simulink subsystem "PROGRAM_COUNTER_06_SS"  (R2022a)
settings: Solver=VariableStepAuto  StartTime=0.0  StopTime=10.0  RelTol=1e-3
libraries: hdlBasic x1928, hlsBasic x1
(part 8 of 12)

== system PROGRAM_COUNTER_06_SS/SUMADOR_64_BITS_00/ALU_SUM_7 ==
  CARRY_IN (1 BIT) : Inport
  A_INPUT (1 BIT) : Inport  Port=2
  B_INPUT (1 BIT) : Inport  Port=3
  Inverter1 : hdlBasic/Inverter  en=off  latency=0  XmcBlockStatus=1  maskContainerNames=group2  block_type=inv  block_config=sysgen:Inverter_config
  Inverter8 : hdlBasic/Inverter  en=off  latency=0  XmcBlockStatus=1  maskContainerNames=group2  block_type=inv  block_config=sysgen:Inverter_config
  Inverter9 : hdlBasic/Inverter  en=off  latency=0  XmcBlockStatus=1  maskContainerNames=group2  block_type=inv  block_config=sysgen:Inverter_config
  Logical : hdlBasic/Logical  logical_function=AND  inputs=2  en=off  latency=0  precision=Full  arith_type=Unsigned  n_bits=16  bin_pt=0  align_bp=on  overflow=[]  quantization=[]  XmcBlockStatus=1  maskContainerNames=tabcontainer1  block_type=logical  block_config=sysgen:Logical_config
  Logical1 : hdlBasic/Logical  logical_function=AND  inputs=2  en=off  latency=0  precision=Full  arith_type=Unsigned  n_bits=16  bin_pt=0  align_bp=on  overflow=[]  quantization=[]  XmcBlockStatus=1  maskContainerNames=tabcontainer1  block_type=logical  block_config=sysgen:Logical_config
  Logical2 : hdlBasic/Logical  logical_function=AND  inputs=2  en=off  latency=0  precision=Full  arith_type=Unsigned  n_bits=16  bin_pt=0  align_bp=on  overflow=[]  quantization=[]  XmcBlockStatus=1  maskContainerNames=tabcontainer1  block_type=logical  block_config=sysgen:Logical_config
  Logical{4..6,9} (4 alike) : hdlBasic/Logical  logical_function=AND  inputs=3  en=off  latency=0  precision=Full  arith_type=Unsigned  n_bits=16  bin_pt=0  align_bp=on  overflow=[]  quantization=[]  XmcBlockStatus=1  maskContainerNames=tabcontainer1  block_type=logical  block_config=sysgen:Logical_config
  Sum : hdlBasic/Logical  logical_function=OR  inputs=4  en=off  latency=0  precision=Full  arith_type=Unsigned  n_bits=16  bin_pt=0  align_bp=on  overflow=[]  quantization=[]  XmcBlockStatus=1  maskContainerNames=tabcontainer1  block_type=logical  block_config=sysgen:Logical_config
  c_out : hdlBasic/Logical  logical_function=OR  inputs=3  en=off  latency=0  precision=Full  arith_type=Unsigned  n_bits=16  bin_pt=0  align_bp=on  overflow=[]  quantization=[]  XmcBlockStatus=1  maskContainerNames=tabcontainer1  block_type=logical  block_config=sysgen:Logical_config
  ALU_OUT (1 BIT) : Outport
  CARRY_OUT (1 BIT) : Outport  Port=2
  wires:
  c_out/1 -> CARRY_OUT (1 BIT)/1
  Logical2/1 -> c_out/3
  Sum/1 -> ALU_OUT (1 BIT)/1
  Inverter9/1 -> Logical4/3, Logical9/3
  Logical5/1 -> Sum/4
  Logical/1 -> c_out/1
  Logical4/1 -> Sum/1
  Logical9/1 -> Sum/2
  Logical6/1 -> Sum/3
  Inverter1/1 -> Logical9/1, Logical6/1
  B_INPUT (1 BIT)/1 -> Inverter9/1, Logical2/2, Logical1/2, Logical6/3, Logical5/3
  CARRY_IN (1 BIT)/1 -> Logical/1, Logical1/1, Logical4/1, Logical5/1, Inverter1/1
  Inverter8/1 -> Logical4/2, Logical6/2
  Logical1/1 -> c_out/2
  A_INPUT (1 BIT)/1 -> Logical9/2, Logical2/1, Logical/2, Logical5/2, Inverter8/1

== system PROGRAM_COUNTER_06_SS/SUMADOR_64_BITS_00/ALU_SUM_8 ==
  CARRY_IN (1 BIT) : Inport
  A_INPUT (1 BIT) : Inport  Port=2
  B_INPUT (1 BIT) : Inport  Port=3
  Inverter1 : hdlBasic/Inverter  en=off  latency=0  XmcBlockStatus=1  maskContainerNames=group2  block_type=inv  block_config=sysgen:Inverter_config
  Inverter8 : hdlBasic/Inverter  en=off  latency=0  XmcBlockStatus=1  maskContainerNames=group2  block_type=inv  block_config=sysgen:Inverter_config
  Inverter9 : hdlBasic/Inverter  en=off  latency=0  XmcBlockStatus=1  maskContainerNames=group2  block_type=inv  block_config=sysgen:Inverter_config
  Logical : hdlBasic/Logical  logical_function=AND  inputs=2  en=off  latency=0  precision=Full  arith_type=Unsigned  n_bits=16  bin_pt=0  align_bp=on  overflow=[]  quantization=[]  XmcBlockStatus=1  maskContainerNames=tabcontainer1  block_type=logical  block_config=sysgen:Logical_config
  Logical1 : hdlBasic/Logical  logical_function=AND  inputs=2  en=off  latency=0  precision=Full  arith_type=Unsigned  n_bits=16  bin_pt=0  align_bp=on  overflow=[]  quantization=[]  XmcBlockStatus=1  maskContainerNames=tabcontainer1  block_type=logical  block_config=sysgen:Logical_config
  Logical2 : hdlBasic/Logical  logical_function=AND  inputs=2  en=off  latency=0  precision=Full  arith_type=Unsigned  n_bits=16  bin_pt=0  align_bp=on  overflow=[]  quantization=[]  XmcBlockStatus=1  maskContainerNames=tabcontainer1  block_type=logical  block_config=sysgen:Logical_config
  Logical{4..6,9} (4 alike) : hdlBasic/Logical  logical_function=AND  inputs=3  en=off  latency=0  precision=Full  arith_type=Unsigned  n_bits=16  bin_pt=0  align_bp=on  overflow=[]  quantization=[]  XmcBlockStatus=1  maskContainerNames=tabcontainer1  block_type=logical  block_config=sysgen:Logical_config
  Sum : hdlBasic/Logical  logical_function=OR  inputs=4  en=off  latency=0  precision=Full  arith_type=Unsigned  n_bits=16  bin_pt=0  align_bp=on  overflow=[]  quantization=[]  XmcBlockStatus=1  maskContainerNames=tabcontainer1  block_type=logical  block_config=sysgen:Logical_config
  c_out : hdlBasic/Logical  logical_function=OR  inputs=3  en=off  latency=0  precision=Full  arith_type=Unsigned  n_bits=16  bin_pt=0  align_bp=on  overflow=[]  quantization=[]  XmcBlockStatus=1  maskContainerNames=tabcontainer1  block_type=logical  block_config=sysgen:Logical_config
  ALU_OUT (1 BIT) : Outport
  CARRY_OUT (1 BIT) : Outport  Port=2
  wires:
  c_out/1 -> CARRY_OUT (1 BIT)/1
  Logical2/1 -> c_out/3
  Sum/1 -> ALU_OUT (1 BIT)/1
  Inverter9/1 -> Logical4/3, Logical9/3
  Logical5/1 -> Sum/4
  Logical/1 -> c_out/1
  Logical4/1 -> Sum/1
  Logical9/1 -> Sum/2
  Logical6/1 -> Sum/3
  Inverter1/1 -> Logical9/1, Logical6/1
  B_INPUT (1 BIT)/1 -> Inverter9/1, Logical2/2, Logical1/2, Logical6/3, Logical5/3
  CARRY_IN (1 BIT)/1 -> Logical/1, Logical1/1, Logical4/1, Logical5/1, Inverter1/1
  Inverter8/1 -> Logical4/2, Logical6/2
  Logical1/1 -> c_out/2
  A_INPUT (1 BIT)/1 -> Logical9/2, Logical2/1, Logical/2, Logical5/2, Inverter8/1

== system PROGRAM_COUNTER_06_SS/SUMADOR_64_BITS_00/ALU_SUM_9 ==
  CARRY_IN (1 BIT) : Inport
  A_INPUT (1 BIT) : Inport  Port=2
  B_INPUT (1 BIT) : Inport  Port=3
  Inverter1 : hdlBasic/Inverter  en=off  latency=0  XmcBlockStatus=1  maskContainerNames=group2  block_type=inv  block_config=sysgen:Inverter_config
  Inverter8 : hdlBasic/Inverter  en=off  latency=0  XmcBlockStatus=1  maskContainerNames=group2  block_type=inv  block_config=sysgen:Inverter_config
  Inverter9 : hdlBasic/Inverter  en=off  latency=0  XmcBlockStatus=1  maskContainerNames=group2  block_type=inv  block_config=sysgen:Inverter_config
  Logical : hdlBasic/Logical  logical_function=AND  inputs=2  en=off  latency=0  precision=Full  arith_type=Unsigned  n_bits=16  bin_pt=0  align_bp=on  overflow=[]  quantization=[]  XmcBlockStatus=1  maskContainerNames=tabcontainer1  block_type=logical  block_config=sysgen:Logical_config
  Logical1 : hdlBasic/Logical  logical_function=AND  inputs=2  en=off  latency=0  precision=Full  arith_type=Unsigned  n_bits=16  bin_pt=0  align_bp=on  overflow=[]  quantization=[]  XmcBlockStatus=1  maskContainerNames=tabcontainer1  block_type=logical  block_config=sysgen:Logical_config
  Logical2 : hdlBasic/Logical  logical_function=AND  inputs=2  en=off  latency=0  precision=Full  arith_type=Unsigned  n_bits=16  bin_pt=0  align_bp=on  overflow=[]  quantization=[]  XmcBlockStatus=1  maskContainerNames=tabcontainer1  block_type=logical  block_config=sysgen:Logical_config
  Logical{4..6,9} (4 alike) : hdlBasic/Logical  logical_function=AND  inputs=3  en=off  latency=0  precision=Full  arith_type=Unsigned  n_bits=16  bin_pt=0  align_bp=on  overflow=[]  quantization=[]  XmcBlockStatus=1  maskContainerNames=tabcontainer1  block_type=logical  block_config=sysgen:Logical_config
  Sum : hdlBasic/Logical  logical_function=OR  inputs=4  en=off  latency=0  precision=Full  arith_type=Unsigned  n_bits=16  bin_pt=0  align_bp=on  overflow=[]  quantization=[]  XmcBlockStatus=1  maskContainerNames=tabcontainer1  block_type=logical  block_config=sysgen:Logical_config
  c_out : hdlBasic/Logical  logical_function=OR  inputs=3  en=off  latency=0  precision=Full  arith_type=Unsigned  n_bits=16  bin_pt=0  align_bp=on  overflow=[]  quantization=[]  XmcBlockStatus=1  maskContainerNames=tabcontainer1  block_type=logical  block_config=sysgen:Logical_config
  ALU_OUT (1 BIT) : Outport
  CARRY_OUT (1 BIT) : Outport  Port=2
  wires:
  c_out/1 -> CARRY_OUT (1 BIT)/1
  Logical2/1 -> c_out/3
  Sum/1 -> ALU_OUT (1 BIT)/1
  Inverter9/1 -> Logical4/3, Logical9/3
  Logical5/1 -> Sum/4
  Logical/1 -> c_out/1
  Logical4/1 -> Sum/1
  Logical9/1 -> Sum/2
  Logical6/1 -> Sum/3
  Inverter1/1 -> Logical9/1, Logical6/1
  B_INPUT (1 BIT)/1 -> Inverter9/1, Logical2/2, Logical1/2, Logical6/3, Logical5/3
  CARRY_IN (1 BIT)/1 -> Logical/1, Logical1/1, Logical4/1, Logical5/1, Inverter1/1
  Inverter8/1 -> Logical4/2, Logical6/2
  Logical1/1 -> c_out/2
  A_INPUT (1 BIT)/1 -> Logical9/2, Logical2/1, Logical/2, Logical5/2, Inverter8/1

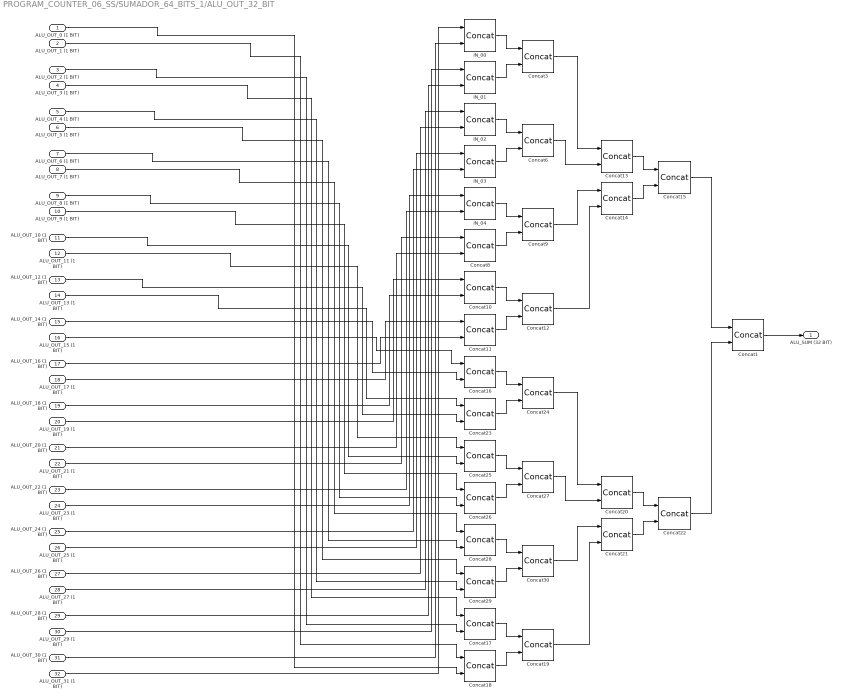
== system PROGRAM_COUNTER_06_SS/SUMADOR_64_BITS_1/ALU_OUT_32_BIT ==
  ALU_OUT_0 (1 BIT) : Inport
  ALU_OUT_1 (1 BIT) : Inport  Port=2
  ALU_OUT_2 (1 BIT) : Inport  Port=3
  ALU_OUT_3 (1 BIT) : Inport  Port=4
  ALU_OUT_4 (1 BIT) : Inport  Port=5
  ALU_OUT_5 (1 BIT) : Inport  Port=6
  ALU_OUT_6 (1 BIT) : Inport  Port=7
  ALU_OUT_7 (1 BIT) : Inport  Port=8
  ALU_OUT_8 (1 BIT) : Inport  Port=9
  ALU_OUT_9 (1 BIT) : Inport  Port=10
  ALU_OUT_10 (1 BIT) : Inport  Port=11
  ALU_OUT_11 (1 BIT) : Inport  Port=12
  ALU_OUT_12 (1 BIT) : Inport  Port=13
  ALU_OUT_13 (1 BIT) : Inport  Port=14
  ALU_OUT_14 (1 BIT) : Inport  Port=15
  ALU_OUT_15 (1 BIT) : Inport  Port=16
  ALU_OUT_16 (1 BIT) : Inport  Port=17
  ALU_OUT_17 (1 BIT) : Inport  Port=18
  ALU_OUT_18 (1 BIT) : Inport  Port=19
  ALU_OUT_19 (1 BIT) : Inport  Port=20
  ALU_OUT_20 (1 BIT) : Inport  Port=21
  ALU_OUT_21 (1 BIT) : Inport  Port=22
  ALU_OUT_22 (1 BIT) : Inport  Port=23
  ALU_OUT_23 (1 BIT) : Inport  Port=24
  ALU_OUT_24 (1 BIT) : Inport  Port=25
  ALU_OUT_25 (1 BIT) : Inport  Port=26
  ALU_OUT_26 (1 BIT) : Inport  Port=27
  ALU_OUT_27 (1 BIT) : Inport  Port=28
  ALU_OUT_28 (1 BIT) : Inport  Port=29
  ALU_OUT_29 (1 BIT) : Inport  Port=30
  ALU_OUT_30 (1 BIT) : Inport  Port=31
  ALU_OUT_31 (1 BIT) : Inport  Port=32
  Concat{1,3,6,8..30} (26 alike) : hdlBasic/Concat  num_inputs=2  XmcBlockStatus=1  maskContainerNames=group1  block_type=concat  block_config=sysgen:Concat_config
  IN_00 : hdlBasic/Concat  num_inputs=2  XmcBlockStatus=1  maskContainerNames=group1  block_type=concat  block_config=sysgen:Concat_config
  IN_01 : hdlBasic/Concat  num_inputs=2  XmcBlockStatus=1  maskContainerNames=group1  block_type=concat  block_config=sysgen:Concat_config
  IN_02 : hdlBasic/Concat  num_inputs=2  XmcBlockStatus=1  maskContainerNames=group1  block_type=concat  block_config=sysgen:Concat_config
  IN_03 : hdlBasic/Concat  num_inputs=2  XmcBlockStatus=1  maskContainerNames=group1  block_type=concat  block_config=sysgen:Concat_config
  IN_04 : hdlBasic/Concat  num_inputs=2  XmcBlockStatus=1  maskContainerNames=group1  block_type=concat  block_config=sysgen:Concat_config
  ALU_SUM (32 BIT) : Outport
  wires:
  ALU_OUT_0 (1 BIT)/1 -> Concat18/2
  ALU_OUT_1 (1 BIT)/1 -> Concat18/1
  ALU_OUT_2 (1 BIT)/1 -> Concat17/2
  ALU_OUT_3 (1 BIT)/1 -> Concat17/1
  ALU_OUT_4 (1 BIT)/1 -> Concat29/2
  ALU_OUT_5 (1 BIT)/1 -> Concat29/1
  ALU_OUT_6 (1 BIT)/1 -> Concat28/2
  ALU_OUT_7 (1 BIT)/1 -> Concat28/1
  ALU_OUT_8 (1 BIT)/1 -> Concat26/2
  ALU_OUT_9 (1 BIT)/1 -> Concat26/1
  ALU_OUT_10 (1 BIT)/1 -> Concat25/2
  ALU_OUT_11 (1 BIT)/1 -> Concat25/1
  ALU_OUT_12 (1 BIT)/1 -> Concat23/2
  ALU_OUT_13 (1 BIT)/1 -> Concat23/1
  ALU_OUT_14 (1 BIT)/1 -> Concat16/2
  ALU_OUT_15 (1 BIT)/1 -> Concat16/1
  ALU_OUT_16 (1 BIT)/1 -> Concat11/2
  ALU_OUT_17 (1 BIT)/1 -> Concat11/1
  ALU_OUT_18 (1 BIT)/1 -> Concat10/2
  ALU_OUT_19 (1 BIT)/1 -> Concat10/1
  ALU_OUT_20 (1 BIT)/1 -> Concat8/2
  ALU_OUT_21 (1 BIT)/1 -> Concat8/1
  ALU_OUT_22 (1 BIT)/1 -> IN_04/2
  ALU_OUT_23 (1 BIT)/1 -> IN_04/1
  ALU_OUT_24 (1 BIT)/1 -> IN_03/2
  ALU_OUT_25 (1 BIT)/1 -> IN_03/1
  ALU_OUT_26 (1 BIT)/1 -> IN_02/2
  ALU_OUT_27 (1 BIT)/1 -> IN_02/1
  ALU_OUT_28 (1 BIT)/1 -> IN_01/2
  ALU_OUT_29 (1 BIT)/1 -> IN_01/1
  ALU_OUT_30 (1 BIT)/1 -> IN_00/2
  ALU_OUT_31 (1 BIT)/1 -> IN_00/1
  Concat1/1 -> ALU_SUM (32 BIT)/1
  Concat12/1 -> Concat14/2
  Concat14/1 -> Concat15/2
  IN_04/1 -> Concat9/1
  Concat8/1 -> Concat9/2
  Concat15/1 -> Concat1/1
  Concat9/1 -> Concat14/1
  IN_03/1 -> Concat6/2
  IN_02/1 -> Concat6/1
  Concat25/1 -> Concat27/1
  Concat18/1 -> Concat19/2
  Concat23/1 -> Concat24/2
  Concat16/1 -> Concat24/1
  Concat24/1 -> Concat20/1
  Concat30/1 -> Concat21/1
  Concat13/1 -> Concat15/1
  Concat6/1 -> Concat13/2
  Concat26/1 -> Concat27/2
  Concat17/1 -> Concat19/1
  Concat20/1 -> Concat22/1
  Concat3/1 -> Concat13/1
  IN_00/1 -> Concat3/1
  Concat21/1 -> Concat22/2
  Concat29/1 -> Concat30/2
  Concat11/1 -> Concat12/2
  Concat28/1 -> Concat30/1
  Concat22/1 -> Concat1/2
  Concat19/1 -> Concat21/2
  Concat27/1 -> Concat20/2
  Concat10/1 -> Concat12/1
  IN_01/1 -> Concat3/2

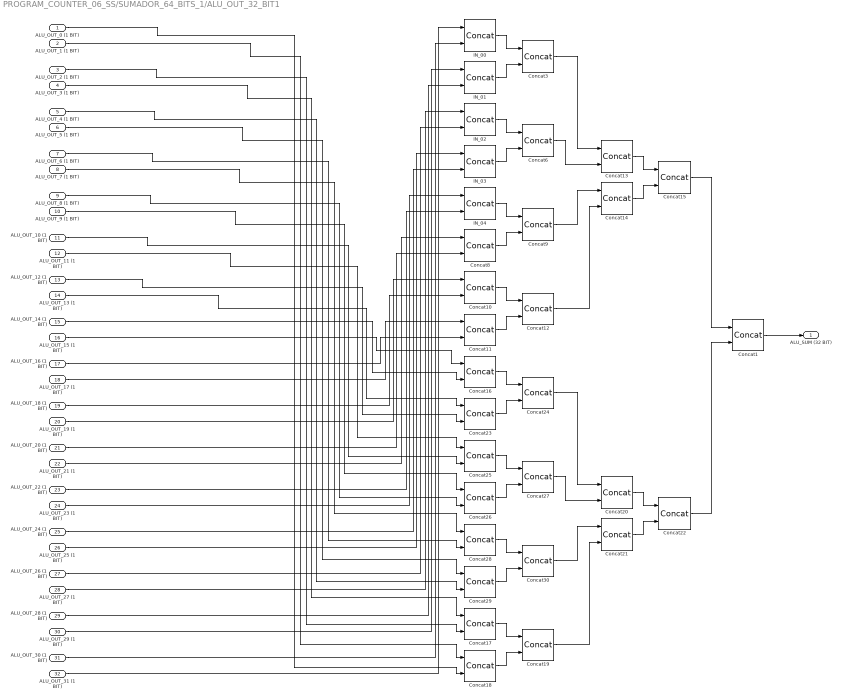
== system PROGRAM_COUNTER_06_SS/SUMADOR_64_BITS_1/ALU_OUT_32_BIT1 ==
  ALU_OUT_0 (1 BIT) : Inport
  ALU_OUT_1 (1 BIT) : Inport  Port=2
  ALU_OUT_2 (1 BIT) : Inport  Port=3
  ALU_OUT_3 (1 BIT) : Inport  Port=4
  ALU_OUT_4 (1 BIT) : Inport  Port=5
  ALU_OUT_5 (1 BIT) : Inport  Port=6
  ALU_OUT_6 (1 BIT) : Inport  Port=7
  ALU_OUT_7 (1 BIT) : Inport  Port=8
  ALU_OUT_8 (1 BIT) : Inport  Port=9
  ALU_OUT_9 (1 BIT) : Inport  Port=10
  ALU_OUT_10 (1 BIT) : Inport  Port=11
  ALU_OUT_11 (1 BIT) : Inport  Port=12
  ALU_OUT_12 (1 BIT) : Inport  Port=13
  ALU_OUT_13 (1 BIT) : Inport  Port=14
  ALU_OUT_14 (1 BIT) : Inport  Port=15
  ALU_OUT_15 (1 BIT) : Inport  Port=16
  ALU_OUT_16 (1 BIT) : Inport  Port=17
  ALU_OUT_17 (1 BIT) : Inport  Port=18
  ALU_OUT_18 (1 BIT) : Inport  Port=19
  ALU_OUT_19 (1 BIT) : Inport  Port=20
  ALU_OUT_20 (1 BIT) : Inport  Port=21
  ALU_OUT_21 (1 BIT) : Inport  Port=22
  ALU_OUT_22 (1 BIT) : Inport  Port=23
  ALU_OUT_23 (1 BIT) : Inport  Port=24
  ALU_OUT_24 (1 BIT) : Inport  Port=25
  ALU_OUT_25 (1 BIT) : Inport  Port=26
  ALU_OUT_26 (1 BIT) : Inport  Port=27
  ALU_OUT_27 (1 BIT) : Inport  Port=28
  ALU_OUT_28 (1 BIT) : Inport  Port=29
  ALU_OUT_29 (1 BIT) : Inport  Port=30
  ALU_OUT_30 (1 BIT) : Inport  Port=31
  ALU_OUT_31 (1 BIT) : Inport  Port=32
  Concat{1,3,6,8..30} (26 alike) : hdlBasic/Concat  num_inputs=2  XmcBlockStatus=1  maskContainerNames=group1  block_type=concat  block_config=sysgen:Concat_config
  IN_00 : hdlBasic/Concat  num_inputs=2  XmcBlockStatus=1  maskContainerNames=group1  block_type=concat  block_config=sysgen:Concat_config
  IN_01 : hdlBasic/Concat  num_inputs=2  XmcBlockStatus=1  maskContainerNames=group1  block_type=concat  block_config=sysgen:Concat_config
  IN_02 : hdlBasic/Concat  num_inputs=2  XmcBlockStatus=1  maskContainerNames=group1  block_type=concat  block_config=sysgen:Concat_config
  IN_03 : hdlBasic/Concat  num_inputs=2  XmcBlockStatus=1  maskContainerNames=group1  block_type=concat  block_config=sysgen:Concat_config
  IN_04 : hdlBasic/Concat  num_inputs=2  XmcBlockStatus=1  maskContainerNames=group1  block_type=concat  block_config=sysgen:Concat_config
  ALU_SUM (32 BIT) : Outport
  wires:
  ALU_OUT_0 (1 BIT)/1 -> Concat18/2
  ALU_OUT_1 (1 BIT)/1 -> Concat18/1
  ALU_OUT_2 (1 BIT)/1 -> Concat17/2
  ALU_OUT_3 (1 BIT)/1 -> Concat17/1
  ALU_OUT_4 (1 BIT)/1 -> Concat29/2
  ALU_OUT_5 (1 BIT)/1 -> Concat29/1
  ALU_OUT_6 (1 BIT)/1 -> Concat28/2
  ALU_OUT_7 (1 BIT)/1 -> Concat28/1
  ALU_OUT_8 (1 BIT)/1 -> Concat26/2
  ALU_OUT_9 (1 BIT)/1 -> Concat26/1
  ALU_OUT_10 (1 BIT)/1 -> Concat25/2
  ALU_OUT_11 (1 BIT)/1 -> Concat25/1
  ALU_OUT_12 (1 BIT)/1 -> Concat23/2
  ALU_OUT_13 (1 BIT)/1 -> Concat23/1
  ALU_OUT_14 (1 BIT)/1 -> Concat16/2
  ALU_OUT_15 (1 BIT)/1 -> Concat16/1
  ALU_OUT_16 (1 BIT)/1 -> Concat11/2
  ALU_OUT_17 (1 BIT)/1 -> Concat11/1
  ALU_OUT_18 (1 BIT)/1 -> Concat10/2
  ALU_OUT_19 (1 BIT)/1 -> Concat10/1
  ALU_OUT_20 (1 BIT)/1 -> Concat8/2
  ALU_OUT_21 (1 BIT)/1 -> Concat8/1
  ALU_OUT_22 (1 BIT)/1 -> IN_04/2
  ALU_OUT_23 (1 BIT)/1 -> IN_04/1
  ALU_OUT_24 (1 BIT)/1 -> IN_03/2
  ALU_OUT_25 (1 BIT)/1 -> IN_03/1
  ALU_OUT_26 (1 BIT)/1 -> IN_02/2
  ALU_OUT_27 (1 BIT)/1 -> IN_02/1
  ALU_OUT_28 (1 BIT)/1 -> IN_01/2
  ALU_OUT_29 (1 BIT)/1 -> IN_01/1
  ALU_OUT_30 (1 BIT)/1 -> IN_00/2
  ALU_OUT_31 (1 BIT)/1 -> IN_00/1
  Concat1/1 -> ALU_SUM (32 BIT)/1
  Concat12/1 -> Concat14/2
  Concat14/1 -> Concat15/2
  IN_04/1 -> Concat9/1
  Concat8/1 -> Concat9/2
  Concat15/1 -> Concat1/1
  Concat9/1 -> Concat14/1
  IN_03/1 -> Concat6/2
  IN_02/1 -> Concat6/1
  Concat25/1 -> Concat27/1
  Concat18/1 -> Concat19/2
  Concat23/1 -> Concat24/2
  Concat16/1 -> Concat24/1
  Concat24/1 -> Concat20/1
  Concat30/1 -> Concat21/1
  Concat13/1 -> Concat15/1
  Concat6/1 -> Concat13/2
  Concat26/1 -> Concat27/2
  Concat17/1 -> Concat19/1
  Concat20/1 -> Concat22/1
  Concat3/1 -> Concat13/1
  IN_00/1 -> Concat3/1
  Concat21/1 -> Concat22/2
  Concat29/1 -> Concat30/2
  Concat11/1 -> Concat12/2
  Concat28/1 -> Concat30/1
  Concat22/1 -> Concat1/2
  Concat19/1 -> Concat21/2
  Concat27/1 -> Concat20/2
  Concat10/1 -> Concat12/1
  IN_01/1 -> Concat3/2

== system PROGRAM_COUNTER_06_SS/SUMADOR_64_BITS_1/ALU_SUM_0 ==
  CARRY_IN (1 BIT) : Inport
  A_INPUT (1 BIT) : Inport  Port=2
  B_INPUT (1 BIT) : Inport  Port=3
  Inverter1 : hdlBasic/Inverter  en=off  latency=0  XmcBlockStatus=1  maskContainerNames=group2  block_type=inv  block_config=sysgen:Inverter_config
  Inverter8 : hdlBasic/Inverter  en=off  latency=0  XmcBlockStatus=1  maskContainerNames=group2  block_type=inv  block_config=sysgen:Inverter_config
  Inverter9 : hdlBasic/Inverter  en=off  latency=0  XmcBlockStatus=1  maskContainerNames=group2  block_type=inv  block_config=sysgen:Inverter_config
  Logical : hdlBasic/Logical  logical_function=AND  inputs=2  en=off  latency=0  precision=Full  arith_type=Unsigned  n_bits=16  bin_pt=0  align_bp=on  overflow=[]  quantization=[]  XmcBlockStatus=1  maskContainerNames=tabcontainer1  block_type=logical  block_config=sysgen:Logical_config
  Logical1 : hdlBasic/Logical  logical_function=AND  inputs=2  en=off  latency=0  precision=Full  arith_type=Unsigned  n_bits=16  bin_pt=0  align_bp=on  overflow=[]  quantization=[]  XmcBlockStatus=1  maskContainerNames=tabcontainer1  block_type=logical  block_config=sysgen:Logical_config
  Logical2 : hdlBasic/Logical  logical_function=AND  inputs=2  en=off  latency=0  precision=Full  arith_type=Unsigned  n_bits=16  bin_pt=0  align_bp=on  overflow=[]  quantization=[]  XmcBlockStatus=1  maskContainerNames=tabcontainer1  block_type=logical  block_config=sysgen:Logical_config
  Logical{4..6,9} (4 alike) : hdlBasic/Logical  logical_function=AND  inputs=3  en=off  latency=0  precision=Full  arith_type=Unsigned  n_bits=16  bin_pt=0  align_bp=on  overflow=[]  quantization=[]  XmcBlockStatus=1  maskContainerNames=tabcontainer1  block_type=logical  block_config=sysgen:Logical_config
  Sum : hdlBasic/Logical  logical_function=OR  inputs=4  en=off  latency=0  precision=Full  arith_type=Unsigned  n_bits=16  bin_pt=0  align_bp=on  overflow=[]  quantization=[]  XmcBlockStatus=1  maskContainerNames=tabcontainer1  block_type=logical  block_config=sysgen:Logical_config
  c_out : hdlBasic/Logical  logical_function=OR  inputs=3  en=off  latency=0  precision=Full  arith_type=Unsigned  n_bits=16  bin_pt=0  align_bp=on  overflow=[]  quantization=[]  XmcBlockStatus=1  maskContainerNames=tabcontainer1  block_type=logical  block_config=sysgen:Logical_config
  ALU_OUT (1 BIT) : Outport
  CARRY_OUT (1 BIT) : Outport  Port=2
  wires:
  c_out/1 -> CARRY_OUT (1 BIT)/1
  Logical2/1 -> c_out/3
  Sum/1 -> ALU_OUT (1 BIT)/1
  Inverter9/1 -> Logical4/3, Logical9/3
  Logical5/1 -> Sum/4
  Logical/1 -> c_out/1
  Logical4/1 -> Sum/1
  Logical9/1 -> Sum/2
  Logical6/1 -> Sum/3
  Inverter1/1 -> Logical9/1, Logical6/1
  B_INPUT (1 BIT)/1 -> Inverter9/1, Logical2/2, Logical1/2, Logical6/3, Logical5/3
  CARRY_IN (1 BIT)/1 -> Logical/1, Logical1/1, Logical4/1, Logical5/1, Inverter1/1
  Inverter8/1 -> Logical4/2, Logical6/2
  Logical1/1 -> c_out/2
  A_INPUT (1 BIT)/1 -> Logical9/2, Logical2/1, Logical/2, Logical5/2, Inverter8/1

== system PROGRAM_COUNTER_06_SS/SUMADOR_64_BITS_1/ALU_SUM_1 ==
  CARRY_IN (1 BIT) : Inport
  A_INPUT (1 BIT) : Inport  Port=2
  B_INPUT (1 BIT) : Inport  Port=3
  Inverter1 : hdlBasic/Inverter  en=off  latency=0  XmcBlockStatus=1  maskContainerNames=group2  block_type=inv  block_config=sysgen:Inverter_config
  Inverter8 : hdlBasic/Inverter  en=off  latency=0  XmcBlockStatus=1  maskContainerNames=group2  block_type=inv  block_config=sysgen:Inverter_config
  Inverter9 : hdlBasic/Inverter  en=off  latency=0  XmcBlockStatus=1  maskContainerNames=group2  block_type=inv  block_config=sysgen:Inverter_config
  Logical : hdlBasic/Logical  logical_function=AND  inputs=2  en=off  latency=0  precision=Full  arith_type=Unsigned  n_bits=16  bin_pt=0  align_bp=on  overflow=[]  quantization=[]  XmcBlockStatus=1  maskContainerNames=tabcontainer1  block_type=logical  block_config=sysgen:Logical_config
  Logical1 : hdlBasic/Logical  logical_function=AND  inputs=2  en=off  latency=0  precision=Full  arith_type=Unsigned  n_bits=16  bin_pt=0  align_bp=on  overflow=[]  quantization=[]  XmcBlockStatus=1  maskContainerNames=tabcontainer1  block_type=logical  block_config=sysgen:Logical_config
  Logical2 : hdlBasic/Logical  logical_function=AND  inputs=2  en=off  latency=0  precision=Full  arith_type=Unsigned  n_bits=16  bin_pt=0  align_bp=on  overflow=[]  quantization=[]  XmcBlockStatus=1  maskContainerNames=tabcontainer1  block_type=logical  block_config=sysgen:Logical_config
  Logical{4..6,9} (4 alike) : hdlBasic/Logical  logical_function=AND  inputs=3  en=off  latency=0  precision=Full  arith_type=Unsigned  n_bits=16  bin_pt=0  align_bp=on  overflow=[]  quantization=[]  XmcBlockStatus=1  maskContainerNames=tabcontainer1  block_type=logical  block_config=sysgen:Logical_config
  Sum : hdlBasic/Logical  logical_function=OR  inputs=4  en=off  latency=0  precision=Full  arith_type=Unsigned  n_bits=16  bin_pt=0  align_bp=on  overflow=[]  quantization=[]  XmcBlockStatus=1  maskContainerNames=tabcontainer1  block_type=logical  block_config=sysgen:Logical_config
  c_out : hdlBasic/Logical  logical_function=OR  inputs=3  en=off  latency=0  precision=Full  arith_type=Unsigned  n_bits=16  bin_pt=0  align_bp=on  overflow=[]  quantization=[]  XmcBlockStatus=1  maskContainerNames=tabcontainer1  block_type=logical  block_config=sysgen:Logical_config
  ALU_OUT (1 BIT) : Outport
  CARRY_OUT (1 BIT) : Outport  Port=2
  wires:
  c_out/1 -> CARRY_OUT (1 BIT)/1
  Logical2/1 -> c_out/3
  Sum/1 -> ALU_OUT (1 BIT)/1
  Inverter9/1 -> Logical4/3, Logical9/3
  Logical5/1 -> Sum/4
  Logical/1 -> c_out/1
  Logical4/1 -> Sum/1
  Logical9/1 -> Sum/2
  Logical6/1 -> Sum/3
  Inverter1/1 -> Logical9/1, Logical6/1
  B_INPUT (1 BIT)/1 -> Inverter9/1, Logical2/2, Logical1/2, Logical6/3, Logical5/3
  CARRY_IN (1 BIT)/1 -> Logical/1, Logical1/1, Logical4/1, Logical5/1, Inverter1/1
  Inverter8/1 -> Logical4/2, Logical6/2
  Logical1/1 -> c_out/2
  A_INPUT (1 BIT)/1 -> Logical9/2, Logical2/1, Logical/2, Logical5/2, Inverter8/1

== system PROGRAM_COUNTER_06_SS/SUMADOR_64_BITS_1/ALU_SUM_10 ==
  CARRY_IN (1 BIT) : Inport
  A_INPUT (1 BIT) : Inport  Port=2
  B_INPUT (1 BIT) : Inport  Port=3
  Inverter1 : hdlBasic/Inverter  en=off  latency=0  XmcBlockStatus=1  maskContainerNames=group2  block_type=inv  block_config=sysgen:Inverter_config
  Inverter8 : hdlBasic/Inverter  en=off  latency=0  XmcBlockStatus=1  maskContainerNames=group2  block_type=inv  block_config=sysgen:Inverter_config
  Inverter9 : hdlBasic/Inverter  en=off  latency=0  XmcBlockStatus=1  maskContainerNames=group2  block_type=inv  block_config=sysgen:Inverter_config
  Logical : hdlBasic/Logical  logical_function=AND  inputs=2  en=off  latency=0  precision=Full  arith_type=Unsigned  n_bits=16  bin_pt=0  align_bp=on  overflow=[]  quantization=[]  XmcBlockStatus=1  maskContainerNames=tabcontainer1  block_type=logical  block_config=sysgen:Logical_config
  Logical1 : hdlBasic/Logical  logical_function=AND  inputs=2  en=off  latency=0  precision=Full  arith_type=Unsigned  n_bits=16  bin_pt=0  align_bp=on  overflow=[]  quantization=[]  XmcBlockStatus=1  maskContainerNames=tabcontainer1  block_type=logical  block_config=sysgen:Logical_config
  Logical2 : hdlBasic/Logical  logical_function=AND  inputs=2  en=off  latency=0  precision=Full  arith_type=Unsigned  n_bits=16  bin_pt=0  align_bp=on  overflow=[]  quantization=[]  XmcBlockStatus=1  maskContainerNames=tabcontainer1  block_type=logical  block_config=sysgen:Logical_config
  Logical{4..6,9} (4 alike) : hdlBasic/Logical  logical_function=AND  inputs=3  en=off  latency=0  precision=Full  arith_type=Unsigned  n_bits=16  bin_pt=0  align_bp=on  overflow=[]  quantization=[]  XmcBlockStatus=1  maskContainerNames=tabcontainer1  block_type=logical  block_config=sysgen:Logical_config
  Sum : hdlBasic/Logical  logical_function=OR  inputs=4  en=off  latency=0  precision=Full  arith_type=Unsigned  n_bits=16  bin_pt=0  align_bp=on  overflow=[]  quantization=[]  XmcBlockStatus=1  maskContainerNames=tabcontainer1  block_type=logical  block_config=sysgen:Logical_config
  c_out : hdlBasic/Logical  logical_function=OR  inputs=3  en=off  latency=0  precision=Full  arith_type=Unsigned  n_bits=16  bin_pt=0  align_bp=on  overflow=[]  quantization=[]  XmcBlockStatus=1  maskContainerNames=tabcontainer1  block_type=logical  block_config=sysgen:Logical_config
  ALU_OUT (1 BIT) : Outport
  CARRY_OUT (1 BIT) : Outport  Port=2
  wires:
  c_out/1 -> CARRY_OUT (1 BIT)/1
  Logical2/1 -> c_out/3
  Sum/1 -> ALU_OUT (1 BIT)/1
  Inverter9/1 -> Logical4/3, Logical9/3
  Logical5/1 -> Sum/4
  Logical/1 -> c_out/1
  Logical4/1 -> Sum/1
  Logical9/1 -> Sum/2
  Logical6/1 -> Sum/3
  Inverter1/1 -> Logical9/1, Logical6/1
  B_INPUT (1 BIT)/1 -> Inverter9/1, Logical2/2, Logical1/2, Logical6/3, Logical5/3
  CARRY_IN (1 BIT)/1 -> Logical/1, Logical1/1, Logical4/1, Logical5/1, Inverter1/1
  Inverter8/1 -> Logical4/2, Logical6/2
  Logical1/1 -> c_out/2
  A_INPUT (1 BIT)/1 -> Logical9/2, Logical2/1, Logical/2, Logical5/2, Inverter8/1

== system PROGRAM_COUNTER_06_SS/SUMADOR_64_BITS_1/ALU_SUM_11 ==
  CARRY_IN (1 BIT) : Inport
  A_INPUT (1 BIT) : Inport  Port=2
  B_INPUT (1 BIT) : Inport  Port=3
  Inverter1 : hdlBasic/Inverter  en=off  latency=0  XmcBlockStatus=1  maskContainerNames=group2  block_type=inv  block_config=sysgen:Inverter_config
  Inverter8 : hdlBasic/Inverter  en=off  latency=0  XmcBlockStatus=1  maskContainerNames=group2  block_type=inv  block_config=sysgen:Inverter_config
  Inverter9 : hdlBasic/Inverter  en=off  latency=0  XmcBlockStatus=1  maskContainerNames=group2  block_type=inv  block_config=sysgen:Inverter_config
  Logical : hdlBasic/Logical  logical_function=AND  inputs=2  en=off  latency=0  precision=Full  arith_type=Unsigned  n_bits=16  bin_pt=0  align_bp=on  overflow=[]  quantization=[]  XmcBlockStatus=1  maskContainerNames=tabcontainer1  block_type=logical  block_config=sysgen:Logical_config
  Logical1 : hdlBasic/Logical  logical_function=AND  inputs=2  en=off  latency=0  precision=Full  arith_type=Unsigned  n_bits=16  bin_pt=0  align_bp=on  overflow=[]  quantization=[]  XmcBlockStatus=1  maskContainerNames=tabcontainer1  block_type=logical  block_config=sysgen:Logical_config
  Logical2 : hdlBasic/Logical  logical_function=AND  inputs=2  en=off  latency=0  precision=Full  arith_type=Unsigned  n_bits=16  bin_pt=0  align_bp=on  overflow=[]  quantization=[]  XmcBlockStatus=1  maskContainerNames=tabcontainer1  block_type=logical  block_config=sysgen:Logical_config
  Logical{4..6,9} (4 alike) : hdlBasic/Logical  logical_function=AND  inputs=3  en=off  latency=0  precision=Full  arith_type=Unsigned  n_bits=16  bin_pt=0  align_bp=on  overflow=[]  quantization=[]  XmcBlockStatus=1  maskContainerNames=tabcontainer1  block_type=logical  block_config=sysgen:Logical_config
  Sum : hdlBasic/Logical  logical_function=OR  inputs=4  en=off  latency=0  precision=Full  arith_type=Unsigned  n_bits=16  bin_pt=0  align_bp=on  overflow=[]  quantization=[]  XmcBlockStatus=1  maskContainerNames=tabcontainer1  block_type=logical  block_config=sysgen:Logical_config
  c_out : hdlBasic/Logical  logical_function=OR  inputs=3  en=off  latency=0  precision=Full  arith_type=Unsigned  n_bits=16  bin_pt=0  align_bp=on  overflow=[]  quantization=[]  XmcBlockStatus=1  maskContainerNames=tabcontainer1  block_type=logical  block_config=sysgen:Logical_config
  ALU_OUT (1 BIT) : Outport
  CARRY_OUT (1 BIT) : Outport  Port=2
  wires:
  c_out/1 -> CARRY_OUT (1 BIT)/1
  Logical2/1 -> c_out/3
  Sum/1 -> ALU_OUT (1 BIT)/1
  Inverter9/1 -> Logical4/3, Logical9/3
  Logical5/1 -> Sum/4
  Logical/1 -> c_out/1
  Logical4/1 -> Sum/1
  Logical9/1 -> Sum/2
  Logical6/1 -> Sum/3
  Inverter1/1 -> Logical9/1, Logical6/1
  B_INPUT (1 BIT)/1 -> Inverter9/1, Logical2/2, Logical1/2, Logical6/3, Logical5/3
  CARRY_IN (1 BIT)/1 -> Logical/1, Logical1/1, Logical4/1, Logical5/1, Inverter1/1
  Inverter8/1 -> Logical4/2, Logical6/2
  Logical1/1 -> c_out/2
  A_INPUT (1 BIT)/1 -> Logical9/2, Logical2/1, Logical/2, Logical5/2, Inverter8/1

== system PROGRAM_COUNTER_06_SS/SUMADOR_64_BITS_1/ALU_SUM_12 ==
  CARRY_IN (1 BIT) : Inport
  A_INPUT (1 BIT) : Inport  Port=2
  B_INPUT (1 BIT) : Inport  Port=3
  Inverter1 : hdlBasic/Inverter  en=off  latency=0  XmcBlockStatus=1  maskContainerNames=group2  block_type=inv  block_config=sysgen:Inverter_config
  Inverter8 : hdlBasic/Inverter  en=off  latency=0  XmcBlockStatus=1  maskContainerNames=group2  block_type=inv  block_config=sysgen:Inverter_config
  Inverter9 : hdlBasic/Inverter  en=off  latency=0  XmcBlockStatus=1  maskContainerNames=group2  block_type=inv  block_config=sysgen:Inverter_config
  Logical : hdlBasic/Logical  logical_function=AND  inputs=2  en=off  latency=0  precision=Full  arith_type=Unsigned  n_bits=16  bin_pt=0  align_bp=on  overflow=[]  quantization=[]  XmcBlockStatus=1  maskContainerNames=tabcontainer1  block_type=logical  block_config=sysgen:Logical_config
  Logical1 : hdlBasic/Logical  logical_function=AND  inputs=2  en=off  latency=0  precision=Full  arith_type=Unsigned  n_bits=16  bin_pt=0  align_bp=on  overflow=[]  quantization=[]  XmcBlockStatus=1  maskContainerNames=tabcontainer1  block_type=logical  block_config=sysgen:Logical_config
  Logical2 : hdlBasic/Logical  logical_function=AND  inputs=2  en=off  latency=0  precision=Full  arith_type=Unsigned  n_bits=16  bin_pt=0  align_bp=on  overflow=[]  quantization=[]  XmcBlockStatus=1  maskContainerNames=tabcontainer1  block_type=logical  block_config=sysgen:Logical_config
  Logical{4..6,9} (4 alike) : hdlBasic/Logical  logical_function=AND  inputs=3  en=off  latency=0  precision=Full  arith_type=Unsigned  n_bits=16  bin_pt=0  align_bp=on  overflow=[]  quantization=[]  XmcBlockStatus=1  maskContainerNames=tabcontainer1  block_type=logical  block_config=sysgen:Logical_config
  Sum : hdlBasic/Logical  logical_function=OR  inputs=4  en=off  latency=0  precision=Full  arith_type=Unsigned  n_bits=16  bin_pt=0  align_bp=on  overflow=[]  quantization=[]  XmcBlockStatus=1  maskContainerNames=tabcontainer1  block_type=logical  block_config=sysgen:Logical_config
  c_out : hdlBasic/Logical  logical_function=OR  inputs=3  en=off  latency=0  precision=Full  arith_type=Unsigned  n_bits=16  bin_pt=0  align_bp=on  overflow=[]  quantization=[]  XmcBlockStatus=1  maskContainerNames=tabcontainer1  block_type=logical  block_config=sysgen:Logical_config
  ALU_OUT (1 BIT) : Outport
  CARRY_OUT (1 BIT) : Outport  Port=2
  wires:
  c_out/1 -> CARRY_OUT (1 BIT)/1
  Logical2/1 -> c_out/3
  Sum/1 -> ALU_OUT (1 BIT)/1
  Inverter9/1 -> Logical4/3, Logical9/3
  Logical5/1 -> Sum/4
  Logical/1 -> c_out/1
  Logical4/1 -> Sum/1
  Logical9/1 -> Sum/2
  Logical6/1 -> Sum/3
  Inverter1/1 -> Logical9/1, Logical6/1
  B_INPUT (1 BIT)/1 -> Inverter9/1, Logical2/2, Logical1/2, Logical6/3, Logical5/3
  CARRY_IN (1 BIT)/1 -> Logical/1, Logical1/1, Logical4/1, Logical5/1, Inverter1/1
  Inverter8/1 -> Logical4/2, Logical6/2
  Logical1/1 -> c_out/2
  A_INPUT (1 BIT)/1 -> Logical9/2, Logical2/1, Logical/2, Logical5/2, Inverter8/1

== system PROGRAM_COUNTER_06_SS/SUMADOR_64_BITS_1/ALU_SUM_13 ==
  CARRY_IN (1 BIT) : Inport
  A_INPUT (1 BIT) : Inport  Port=2
  B_INPUT (1 BIT) : Inport  Port=3
  Inverter1 : hdlBasic/Inverter  en=off  latency=0  XmcBlockStatus=1  maskContainerNames=group2  block_type=inv  block_config=sysgen:Inverter_config
  Inverter8 : hdlBasic/Inverter  en=off  latency=0  XmcBlockStatus=1  maskContainerNames=group2  block_type=inv  block_config=sysgen:Inverter_config
  Inverter9 : hdlBasic/Inverter  en=off  latency=0  XmcBlockStatus=1  maskContainerNames=group2  block_type=inv  block_config=sysgen:Inverter_config
  Logical : hdlBasic/Logical  logical_function=AND  inputs=2  en=off  latency=0  precision=Full  arith_type=Unsigned  n_bits=16  bin_pt=0  align_bp=on  overflow=[]  quantization=[]  XmcBlockStatus=1  maskContainerNames=tabcontainer1  block_type=logical  block_config=sysgen:Logical_config
  Logical1 : hdlBasic/Logical  logical_function=AND  inputs=2  en=off  latency=0  precision=Full  arith_type=Unsigned  n_bits=16  bin_pt=0  align_bp=on  overflow=[]  quantization=[]  XmcBlockStatus=1  maskContainerNames=tabcontainer1  block_type=logical  block_config=sysgen:Logical_config
  Logical2 : hdlBasic/Logical  logical_function=AND  inputs=2  en=off  latency=0  precision=Full  arith_type=Unsigned  n_bits=16  bin_pt=0  align_bp=on  overflow=[]  quantization=[]  XmcBlockStatus=1  maskContainerNames=tabcontainer1  block_type=logical  block_config=sysgen:Logical_config
  Logical{4..6,9} (4 alike) : hdlBasic/Logical  logical_function=AND  inputs=3  en=off  latency=0  precision=Full  arith_type=Unsigned  n_bits=16  bin_pt=0  align_bp=on  overflow=[]  quantization=[]  XmcBlockStatus=1  maskContainerNames=tabcontainer1  block_type=logical  block_config=sysgen:Logical_config
  Sum : hdlBasic/Logical  logical_function=OR  inputs=4  en=off  latency=0  precision=Full  arith_type=Unsigned  n_bits=16  bin_pt=0  align_bp=on  overflow=[]  quantization=[]  XmcBlockStatus=1  maskContainerNames=tabcontainer1  block_type=logical  block_config=sysgen:Logical_config
  c_out : hdlBasic/Logical  logical_function=OR  inputs=3  en=off  latency=0  precision=Full  arith_type=Unsigned  n_bits=16  bin_pt=0  align_bp=on  overflow=[]  quantization=[]  XmcBlockStatus=1  maskContainerNames=tabcontainer1  block_type=logical  block_config=sysgen:Logical_config
  ALU_OUT (1 BIT) : Outport
  CARRY_OUT (1 BIT) : Outport  Port=2
  wires:
  c_out/1 -> CARRY_OUT (1 BIT)/1
  Logical2/1 -> c_out/3
  Sum/1 -> ALU_OUT (1 BIT)/1
  Inverter9/1 -> Logical4/3, Logical9/3
  Logical5/1 -> Sum/4
  Logical/1 -> c_out/1
  Logical4/1 -> Sum/1
  Logical9/1 -> Sum/2
  Logical6/1 -> Sum/3
  Inverter1/1 -> Logical9/1, Logical6/1
  B_INPUT (1 BIT)/1 -> Inverter9/1, Logical2/2, Logical1/2, Logical6/3, Logical5/3
  CARRY_IN (1 BIT)/1 -> Logical/1, Logical1/1, Logical4/1, Logical5/1, Inverter1/1
  Inverter8/1 -> Logical4/2, Logical6/2
  Logical1/1 -> c_out/2
  A_INPUT (1 BIT)/1 -> Logical9/2, Logical2/1, Logical/2, Logical5/2, Inverter8/1

== system PROGRAM_COUNTER_06_SS/SUMADOR_64_BITS_1/ALU_SUM_14 ==
  CARRY_IN (1 BIT) : Inport
  A_INPUT (1 BIT) : Inport  Port=2
  B_INPUT (1 BIT) : Inport  Port=3
  Inverter1 : hdlBasic/Inverter  en=off  latency=0  XmcBlockStatus=1  maskContainerNames=group2  block_type=inv  block_config=sysgen:Inverter_config
  Inverter8 : hdlBasic/Inverter  en=off  latency=0  XmcBlockStatus=1  maskContainerNames=group2  block_type=inv  block_config=sysgen:Inverter_config
  Inverter9 : hdlBasic/Inverter  en=off  latency=0  XmcBlockStatus=1  maskContainerNames=group2  block_type=inv  block_config=sysgen:Inverter_config
  Logical : hdlBasic/Logical  logical_function=AND  inputs=2  en=off  latency=0  precision=Full  arith_type=Unsigned  n_bits=16  bin_pt=0  align_bp=on  overflow=[]  quantization=[]  XmcBlockStatus=1  maskContainerNames=tabcontainer1  block_type=logical  block_config=sysgen:Logical_config
  Logical1 : hdlBasic/Logical  logical_function=AND  inputs=2  en=off  latency=0  precision=Full  arith_type=Unsigned  n_bits=16  bin_pt=0  align_bp=on  overflow=[]  quantization=[]  XmcBlockStatus=1  maskContainerNames=tabcontainer1  block_type=logical  block_config=sysgen:Logical_config
  Logical2 : hdlBasic/Logical  logical_function=AND  inputs=2  en=off  latency=0  precision=Full  arith_type=Unsigned  n_bits=16  bin_pt=0  align_bp=on  overflow=[]  quantization=[]  XmcBlockStatus=1  maskContainerNames=tabcontainer1  block_type=logical  block_config=sysgen:Logical_config
  Logical{4..6,9} (4 alike) : hdlBasic/Logical  logical_function=AND  inputs=3  en=off  latency=0  precision=Full  arith_type=Unsigned  n_bits=16  bin_pt=0  align_bp=on  overflow=[]  quantization=[]  XmcBlockStatus=1  maskContainerNames=tabcontainer1  block_type=logical  block_config=sysgen:Logical_config
  Sum : hdlBasic/Logical  logical_function=OR  inputs=4  en=off  latency=0  precision=Full  arith_type=Unsigned  n_bits=16  bin_pt=0  align_bp=on  overflow=[]  quantization=[]  XmcBlockStatus=1  maskContainerNames=tabcontainer1  block_type=logical  block_config=sysgen:Logical_config
  c_out : hdlBasic/Logical  logical_function=OR  inputs=3  en=off  latency=0  precision=Full  arith_type=Unsigned  n_bits=16  bin_pt=0  align_bp=on  overflow=[]  quantization=[]  XmcBlockStatus=1  maskContainerNames=tabcontainer1  block_type=logical  block_config=sysgen:Logical_config
  ALU_OUT (1 BIT) : Outport
  CARRY_OUT (1 BIT) : Outport  Port=2
  wires:
  c_out/1 -> CARRY_OUT (1 BIT)/1
  Logical2/1 -> c_out/3
  Sum/1 -> ALU_OUT (1 BIT)/1
  Inverter9/1 -> Logical4/3, Logical9/3
  Logical5/1 -> Sum/4
  Logical/1 -> c_out/1
  Logical4/1 -> Sum/1
  Logical9/1 -> Sum/2
  Logical6/1 -> Sum/3
  Inverter1/1 -> Logical9/1, Logical6/1
  B_INPUT (1 BIT)/1 -> Inverter9/1, Logical2/2, Logical1/2, Logical6/3, Logical5/3
  CARRY_IN (1 BIT)/1 -> Logical/1, Logical1/1, Logical4/1, Logical5/1, Inverter1/1
  Inverter8/1 -> Logical4/2, Logical6/2
  Logical1/1 -> c_out/2
  A_INPUT (1 BIT)/1 -> Logical9/2, Logical2/1, Logical/2, Logical5/2, Inverter8/1

== system PROGRAM_COUNTER_06_SS/SUMADOR_64_BITS_1/ALU_SUM_15 ==
  CARRY_IN (1 BIT) : Inport
  A_INPUT (1 BIT) : Inport  Port=2
  B_INPUT (1 BIT) : Inport  Port=3
  Inverter1 : hdlBasic/Inverter  en=off  latency=0  XmcBlockStatus=1  maskContainerNames=group2  block_type=inv  block_config=sysgen:Inverter_config
  Inverter8 : hdlBasic/Inverter  en=off  latency=0  XmcBlockStatus=1  maskContainerNames=group2  block_type=inv  block_config=sysgen:Inverter_config
  Inverter9 : hdlBasic/Inverter  en=off  latency=0  XmcBlockStatus=1  maskContainerNames=group2  block_type=inv  block_config=sysgen:Inverter_config
  Logical : hdlBasic/Logical  logical_function=AND  inputs=2  en=off  latency=0  precision=Full  arith_type=Unsigned  n_bits=16  bin_pt=0  align_bp=on  overflow=[]  quantization=[]  XmcBlockStatus=1  maskContainerNames=tabcontainer1  block_type=logical  block_config=sysgen:Logical_config
  Logical1 : hdlBasic/Logical  logical_function=AND  inputs=2  en=off  latency=0  precision=Full  arith_type=Unsigned  n_bits=16  bin_pt=0  align_bp=on  overflow=[]  quantization=[]  XmcBlockStatus=1  maskContainerNames=tabcontainer1  block_type=logical  block_config=sysgen:Logical_config
  Logical2 : hdlBasic/Logical  logical_function=AND  inputs=2  en=off  latency=0  precision=Full  arith_type=Unsigned  n_bits=16  bin_pt=0  align_bp=on  overflow=[]  quantization=[]  XmcBlockStatus=1  maskContainerNames=tabcontainer1  block_type=logical  block_config=sysgen:Logical_config
  Logical{4..6,9} (4 alike) : hdlBasic/Logical  logical_function=AND  inputs=3  en=off  latency=0  precision=Full  arith_type=Unsigned  n_bits=16  bin_pt=0  align_bp=on  overflow=[]  quantization=[]  XmcBlockStatus=1  maskContainerNames=tabcontainer1  block_type=logical  block_config=sysgen:Logical_config
  Sum : hdlBasic/Logical  logical_function=OR  inputs=4  en=off  latency=0  precision=Full  arith_type=Unsigned  n_bits=16  bin_pt=0  align_bp=on  overflow=[]  quantization=[]  XmcBlockStatus=1  maskContainerNames=tabcontainer1  block_type=logical  block_config=sysgen:Logical_config
  c_out : hdlBasic/Logical  logical_function=OR  inputs=3  en=off  latency=0  precision=Full  arith_type=Unsigned  n_bits=16  bin_pt=0  align_bp=on  overflow=[]  quantization=[]  XmcBlockStatus=1  maskContainerNames=tabcontainer1  block_type=logical  block_config=sysgen:Logical_config
  ALU_OUT (1 BIT) : Outport
  CARRY_OUT (1 BIT) : Outport  Port=2
  wires:
  c_out/1 -> CARRY_OUT (1 BIT)/1
  Logical2/1 -> c_out/3
  Sum/1 -> ALU_OUT (1 BIT)/1
  Inverter9/1 -> Logical4/3, Logical9/3
  Logical5/1 -> Sum/4
  Logical/1 -> c_out/1
  Logical4/1 -> Sum/1
  Logical9/1 -> Sum/2
  Logical6/1 -> Sum/3
  Inverter1/1 -> Logical9/1, Logical6/1
  B_INPUT (1 BIT)/1 -> Inverter9/1, Logical2/2, Logical1/2, Logical6/3, Logical5/3
  CARRY_IN (1 BIT)/1 -> Logical/1, Logical1/1, Logical4/1, Logical5/1, Inverter1/1
  Inverter8/1 -> Logical4/2, Logical6/2
  Logical1/1 -> c_out/2
  A_INPUT (1 BIT)/1 -> Logical9/2, Logical2/1, Logical/2, Logical5/2, Inverter8/1

== system PROGRAM_COUNTER_06_SS/SUMADOR_64_BITS_1/ALU_SUM_16 ==
  CARRY_IN (1 BIT) : Inport
  A_INPUT (1 BIT) : Inport  Port=2
  B_INPUT (1 BIT) : Inport  Port=3
  Inverter1 : hdlBasic/Inverter  en=off  latency=0  XmcBlockStatus=1  maskContainerNames=group2  block_type=inv  block_config=sysgen:Inverter_config
  Inverter8 : hdlBasic/Inverter  en=off  latency=0  XmcBlockStatus=1  maskContainerNames=group2  block_type=inv  block_config=sysgen:Inverter_config
  Inverter9 : hdlBasic/Inverter  en=off  latency=0  XmcBlockStatus=1  maskContainerNames=group2  block_type=inv  block_config=sysgen:Inverter_config
  Logical : hdlBasic/Logical  logical_function=AND  inputs=2  en=off  latency=0  precision=Full  arith_type=Unsigned  n_bits=16  bin_pt=0  align_bp=on  overflow=[]  quantization=[]  XmcBlockStatus=1  maskContainerNames=tabcontainer1  block_type=logical  block_config=sysgen:Logical_config
  Logical1 : hdlBasic/Logical  logical_function=AND  inputs=2  en=off  latency=0  precision=Full  arith_type=Unsigned  n_bits=16  bin_pt=0  align_bp=on  overflow=[]  quantization=[]  XmcBlockStatus=1  maskContainerNames=tabcontainer1  block_type=logical  block_config=sysgen:Logical_config
  Logical2 : hdlBasic/Logical  logical_function=AND  inputs=2  en=off  latency=0  precision=Full  arith_type=Unsigned  n_bits=16  bin_pt=0  align_bp=on  overflow=[]  quantization=[]  XmcBlockStatus=1  maskContainerNames=tabcontainer1  block_type=logical  block_config=sysgen:Logical_config
  Logical{4..6,9} (4 alike) : hdlBasic/Logical  logical_function=AND  inputs=3  en=off  latency=0  precision=Full  arith_type=Unsigned  n_bits=16  bin_pt=0  align_bp=on  overflow=[]  quantization=[]  XmcBlockStatus=1  maskContainerNames=tabcontainer1  block_type=logical  block_config=sysgen:Logical_config
  Sum : hdlBasic/Logical  logical_function=OR  inputs=4  en=off  latency=0  precision=Full  arith_type=Unsigned  n_bits=16  bin_pt=0  align_bp=on  overflow=[]  quantization=[]  XmcBlockStatus=1  maskContainerNames=tabcontainer1  block_type=logical  block_config=sysgen:Logical_config
  c_out : hdlBasic/Logical  logical_function=OR  inputs=3  en=off  latency=0  precision=Full  arith_type=Unsigned  n_bits=16  bin_pt=0  align_bp=on  overflow=[]  quantization=[]  XmcBlockStatus=1  maskContainerNames=tabcontainer1  block_type=logical  block_config=sysgen:Logical_config
  ALU_OUT (1 BIT) : Outport
  CARRY_OUT (1 BIT) : Outport  Port=2
  wires:
  c_out/1 -> CARRY_OUT (1 BIT)/1
  Logical2/1 -> c_out/3
  Sum/1 -> ALU_OUT (1 BIT)/1
  Inverter9/1 -> Logical4/3, Logical9/3
  Logical5/1 -> Sum/4
  Logical/1 -> c_out/1
  Logical4/1 -> Sum/1
  Logical9/1 -> Sum/2
  Logical6/1 -> Sum/3
  Inverter1/1 -> Logical9/1, Logical6/1
  B_INPUT (1 BIT)/1 -> Inverter9/1, Logical2/2, Logical1/2, Logical6/3, Logical5/3
  CARRY_IN (1 BIT)/1 -> Logical/1, Logical1/1, Logical4/1, Logical5/1, Inverter1/1
  Inverter8/1 -> Logical4/2, Logical6/2
  Logical1/1 -> c_out/2
  A_INPUT (1 BIT)/1 -> Logical9/2, Logical2/1, Logical/2, Logical5/2, Inverter8/1

== system PROGRAM_COUNTER_06_SS/SUMADOR_64_BITS_1/ALU_SUM_17 ==
  CARRY_IN (1 BIT) : Inport
  A_INPUT (1 BIT) : Inport  Port=2
  B_INPUT (1 BIT) : Inport  Port=3
  Inverter1 : hdlBasic/Inverter  en=off  latency=0  XmcBlockStatus=1  maskContainerNames=group2  block_type=inv  block_config=sysgen:Inverter_config
  Inverter8 : hdlBasic/Inverter  en=off  latency=0  XmcBlockStatus=1  maskContainerNames=group2  block_type=inv  block_config=sysgen:Inverter_config
  Inverter9 : hdlBasic/Inverter  en=off  latency=0  XmcBlockStatus=1  maskContainerNames=group2  block_type=inv  block_config=sysgen:Inverter_config
  Logical : hdlBasic/Logical  logical_function=AND  inputs=2  en=off  latency=0  precision=Full  arith_type=Unsigned  n_bits=16  bin_pt=0  align_bp=on  overflow=[]  quantization=[]  XmcBlockStatus=1  maskContainerNames=tabcontainer1  block_type=logical  block_config=sysgen:Logical_config
  Logical1 : hdlBasic/Logical  logical_function=AND  inputs=2  en=off  latency=0  precision=Full  arith_type=Unsigned  n_bits=16  bin_pt=0  align_bp=on  overflow=[]  quantization=[]  XmcBlockStatus=1  maskContainerNames=tabcontainer1  block_type=logical  block_config=sysgen:Logical_config
  Logical2 : hdlBasic/Logical  logical_function=AND  inputs=2  en=off  latency=0  precision=Full  arith_type=Unsigned  n_bits=16  bin_pt=0  align_bp=on  overflow=[]  quantization=[]  XmcBlockStatus=1  maskContainerNames=tabcontainer1  block_type=logical  block_config=sysgen:Logical_config
  Logical{4..6,9} (4 alike) : hdlBasic/Logical  logical_function=AND  inputs=3  en=off  latency=0  precision=Full  arith_type=Unsigned  n_bits=16  bin_pt=0  align_bp=on  overflow=[]  quantization=[]  XmcBlockStatus=1  maskContainerNames=tabcontainer1  block_type=logical  block_config=sysgen:Logical_config
  Sum : hdlBasic/Logical  logical_function=OR  inputs=4  en=off  latency=0  precision=Full  arith_type=Unsigned  n_bits=16  bin_pt=0  align_bp=on  overflow=[]  quantization=[]  XmcBlockStatus=1  maskContainerNames=tabcontainer1  block_type=logical  block_config=sysgen:Logical_config
  c_out : hdlBasic/Logical  logical_function=OR  inputs=3  en=off  latency=0  precision=Full  arith_type=Unsigned  n_bits=16  bin_pt=0  align_bp=on  overflow=[]  quantization=[]  XmcBlockStatus=1  maskContainerNames=tabcontainer1  block_type=logical  block_config=sysgen:Logical_config
  ALU_OUT (1 BIT) : Outport
  CARRY_OUT (1 BIT) : Outport  Port=2
  wires:
  c_out/1 -> CARRY_OUT (1 BIT)/1
  Logical2/1 -> c_out/3
  Sum/1 -> ALU_OUT (1 BIT)/1
  Inverter9/1 -> Logical4/3, Logical9/3
  Logical5/1 -> Sum/4
  Logical/1 -> c_out/1
  Logical4/1 -> Sum/1
  Logical9/1 -> Sum/2
  Logical6/1 -> Sum/3
  Inverter1/1 -> Logical9/1, Logical6/1
  B_INPUT (1 BIT)/1 -> Inverter9/1, Logical2/2, Logical1/2, Logical6/3, Logical5/3
  CARRY_IN (1 BIT)/1 -> Logical/1, Logical1/1, Logical4/1, Logical5/1, Inverter1/1
  Inverter8/1 -> Logical4/2, Logical6/2
  Logical1/1 -> c_out/2
  A_INPUT (1 BIT)/1 -> Logical9/2, Logical2/1, Logical/2, Logical5/2, Inverter8/1
